simulink model "call_V_solve"  (R2019a)
settings: Solver=FixedStepAuto  StartTime=0.0  StopTime=10.0  MaxStep=0.2  RelTol=1e-3
undefined symbols (not defined in the file or in its folder): x0_nom
settings Model: Creator=ztakeo  LastModifiedBy=ztakeo

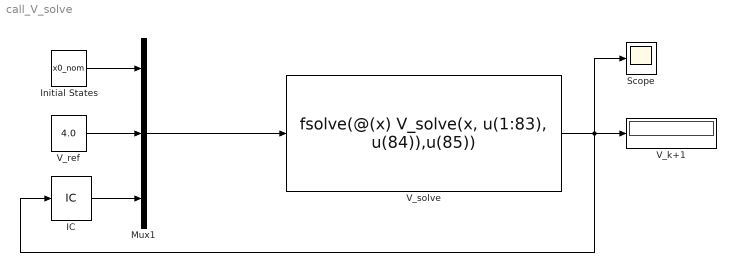
== system call_V_solve ==
  IC : InitialCondition
  Initial States : Constant  Value=x0_nom
  Mux1 : Mux  Inputs=3
  Scope : Scope
  V_k+1 : Display
  "V_ref " : Constant  Value=4.0
  V_solve : MATLABFcn  MATLABFcn=fsolve(@(x) V_solve(x, u(1:83), u(84)),u(85))  OutputDimensions=1
  wires:
  Initial States/1 -> Mux1/1
  "V_ref "/1 -> Mux1/2
  IC/1 -> Mux1/3
  Mux1/1 -> V_solve/1
  V_solve/1 -> IC/1, Scope/1, V_k+1/1
